simulink model "magball_validate_nonlinear"  (Simulink 7.6)
settings: Solver=ode45  StartTime=0.0  StopTime=10  RelTol=1e-3
model workspace (MAT data in the model file):
  op_magball_validate_nonlinear : opcond.OperatingPoint (value not decoded)
PreLoadFcn:
  | magballdat
  | magballop
values from neighbouring files (symbols this model uses):
  beta = 0.001    [magballdat.m]
  L = 0.02    [magballdat.m]    (also in scd_aero_guid_dat.m = 0.0065; scdaircraftpad.m = LinearAircraft.values(:,:,17); scdsaturationDFpad.m = zpk([],[0 -1 -10],1))
  m = 0.1    [magballdat.m]
  R = 2    [magballdat.m]    (also in scd_aero_guid_dat.m = 287.26; scdboilerpad.m = diag([1e2,1e6]); scddcmotorpad.m = [2,1.8,2.2])
settings Model: Creator=The MathWorks Inc.  BufferReuse=off
settings SolverCC: InsertRTBMode=Auto
settings DataIOCC: ExternalInput=getinputstruct(op_magball_validate_nonlinear)  InitialState=getstatestruct(op_magball_validate_nonlinear)  LoadExternalInput=on  LoadInitialState=on  SignalLoggingName=logsOut
settings OptimizationCC: BlockReduction=off  InlineParams=on  InlineInvariantSignals=on  BufferReuse=off  InitFltsAndDblsToZero=on
settings DebuggingCC: SaveWithParameterizedLinksMsg=none  SignalResolutionControl=TryResolveAllWithWarning  SolverPrmCheckMsg=none  MultiTaskDSMMsg=warning  StrictBusMsg=None
settings HardwareCC: TargetUnknown=on
settings CodeAppCC: CustomSymbolStrFcn=$F$N$M
settings GRTTargetCC: TargetFcnLib=ansi_tfl_tmw.mat

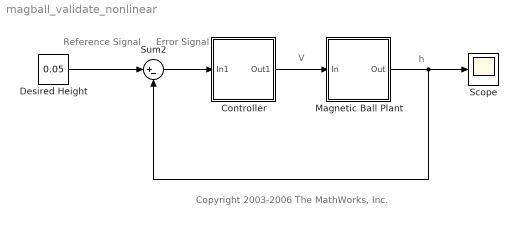
== system magball_validate_nonlinear ==
  note: Error
      | Signal
  note: Reference
      | Signal
  note: V
  note: h
  note: Copyright 2003-2006 The MathWorks, Inc.
  Controller : Subsystem
      settings: RTWMemSecFuncInitTerm=Default  RTWMemSecFuncExecute=Default  RTWMemSecDataConstants=Default  RTWMemSecDataInternal=Default  RTWMemSecDataParameters=Default
  Desired Height : Constant  Value=0.05
  Magnetic Ball Plant : Subsystem
      settings: RTWMemSecFuncInitTerm=Default  RTWMemSecFuncExecute=Default  RTWMemSecDataConstants=Default  RTWMemSecDataInternal=Default  RTWMemSecDataParameters=Default
  Scope : Scope
  Sum2 : Sum  Inputs=|+-
  wires:
  Magnetic Ball Plant/1(Out) -> Scope/1, Sum2/2
  Sum2/1 -> Controller/1(In1)
  Controller/1(Out1) -> Magnetic Ball Plant/1(In)
  Desired Height/1 -> Sum2/1

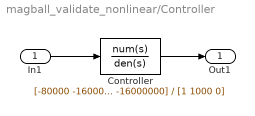
== system magball_validate_nonlinear/Controller ==
  In1 : Inport
  Controller : TransferFcn  Numerator=[-80000 -1600000 -16000000]  Denominator=[1 1000 0]
  Out1 : Outport
  wires:
  In1/1 -> Controller/1
  Controller/1 -> Out1/1

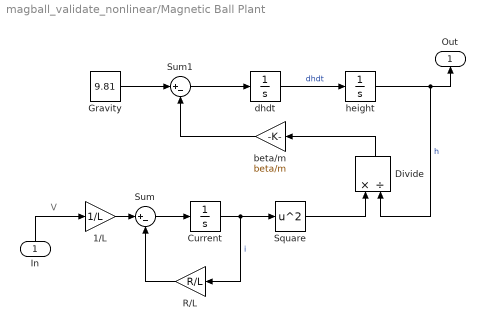
== system magball_validate_nonlinear/Magnetic Ball Plant ==
  note: V
  In : Inport
  1/L : Gain  Gain=1/L
  Current : Integrator  InitialCondition=7.0036
  Divide : Product  Inputs=*/
  Gravity : Constant  Value=9.81
  R/L : Gain  Gain=R/L
  Square : Math  Operator=square  SaturateOnIntegerOverflow=on
  Sum : Sum  Inputs=|+-
  Sum1 : Sum  Inputs=|+-
  beta/m : Gain  Gain=beta/m
  dhdt : Integrator
  height : Integrator  InitialCondition=0.05
  Out : Outport
  wires:
  dhdt/1 -> height/1  "dhdt"
  height/1 -> Out/1, Divide/2  "h"
  Sum/1 -> Current/1
  1/L/1 -> Sum/1
  R/L/1 -> Sum/2
  Current/1 -> Square/1, R/L/1  "i"
  Square/1 -> Divide/1
  Divide/1 -> beta/m/1
  Gravity/1 -> Sum1/1
  beta/m/1 -> Sum1/2
  Sum1/1 -> dhdt/1
  In/1 -> 1/L/1
